simulink model "modelo_geral"  (R2015a)
settings: Solver=ode1  SolverMode=SingleTasking  StartTime=0.0  StopTime=10  FixedStep=0.01  RelTol=1e-3
values from neighbouring files (symbols this model uses):
  K = 54.96    [exp11.m]
  KNL = 59.7881    [exp11.m]
  Kp = 1.604    [exp11.m]
  Kpi = 0.5    [exp11.m]
  Kt = KtL    (= 0.0169213973799)    [exp11.m]
  T = 0.27    [exp11.m]
  U = Kp*pi/2    (= 2.51955730818)    [exp11.m]
undefined symbols (not defined in the file): phi
settings Model: CovExternalEMLEnable=on  Creator=rpm  LastModifiedBy=caiod
settings DataIOCC: LimitDataPoints=off  SignalLoggingSaveFormat=ModelDataLogs  SaveOutput=off  SignalLogging=off  DSMLogging=off  SaveTime=off  TimeSaveName=t
settings OptimizationCC: ExpressionDepthLimit=2147483647  InitFltsAndDblsToZero=on
settings DebuggingCC: UnderspecifiedInitializationDetection=Classic  MergeDetectMultiDrivingBlocksExec=none  FcnCallInpInsideContextMsg=EnableAllAsWarning  StateNameClashWarn=warning
settings GRTTargetCC: CombineOutputUpdateFcns=off  GRTInterface=on

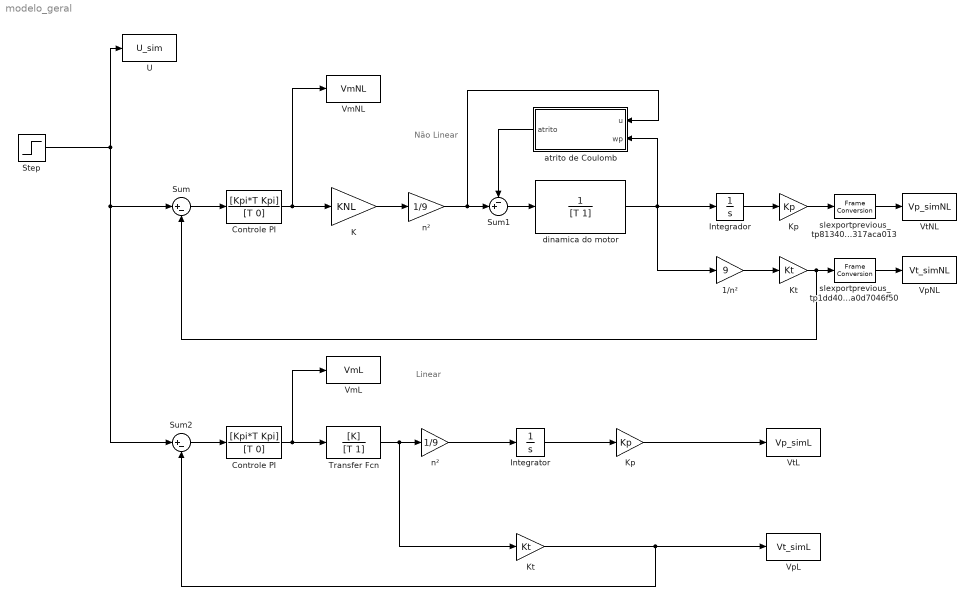
== system modelo_geral ==
  note: Não
      | Linear
  note: Linear
  " VpNL" : ToWorkspace  VariableName=Vt_simNL  SaveFormat=Timeseries  SampleTime=-1
  1/n² : Gain  Gain=9
  Controle PI : TransferFcn  Numerator=[Kpi*T Kpi]  Denominator=[T 0]
  "Controle PI " : TransferFcn  Numerator=[Kpi*T Kpi]  Denominator=[T 0]
  Integrador : Integrator
  Integrator : Integrator
  K : Gain  Gain=KNL
  Kp : Gain  Gain=Kp
  "Kp " : Gain  Gain=Kp
  Kt : Gain  Gain=Kt
  "Kt " : Gain  Gain=Kt
  Step : Step  After=U  SampleTime=0
  Sum : Sum  Inputs=|+-
  Sum1 : Sum  Inputs=-+|
  Sum2 : Sum  Inputs=|+-
  Transfer Fcn : TransferFcn  Numerator=[K]  Denominator=[T 1]
  U : ToWorkspace  VariableName=U_sim  SaveFormat=Timeseries  SampleTime=-1
  "VmL " : ToWorkspace  VariableName=VmL  SaveFormat=Timeseries  SampleTime=-1
  "VmNL " : ToWorkspace  VariableName=VmNL  SaveFormat=Timeseries  SampleTime=-1
  "VpL " : ToWorkspace  VariableName=Vt_simL  SaveFormat=Timeseries  SampleTime=-1
  VtL : ToWorkspace  VariableName=Vp_simL  SaveFormat=Timeseries  SampleTime=-1
  VtNL : ToWorkspace  VariableName=Vp_simNL  SaveFormat=Timeseries  SampleTime=-1
  atrito de Coulomb : Subsystem  mask{phi=phi}
      mask Display: fprintf('phi = %3.1f', phi)
  dinamica do motor : TransferFcn  Denominator=[T 1]
  n² : Gain  Gain=1/9
  "n² " : Gain  Gain=1/9
  slexportprevious_tp1dd40cb0_336a_46da_8b79_bfa0d7046f50 : FrameConversion  OutFrame=Sample-based
  slexportprevious_tp8134031d_9c58_445d_bef1_a0d317aca013 : FrameConversion  OutFrame=Sample-based
  wires:
  dinamica do motor/1 -> 1/n²/1, Integrador/1, atrito de Coulomb/2(wp)
  Integrador/1 -> Kp/1
  K/1 -> n²/1
  n²/1 -> atrito de Coulomb/1(u), Sum1/2
  atrito de Coulomb/1(atrito) -> Sum1/1
  Sum1/1 -> dinamica do motor/1
  1/n²/1 -> Kt/1
  slexportprevious_tp1dd40cb0_336a_46da_8b79_bfa0d7046f50/1 -> " VpNL"/1
  Kp/1 -> slexportprevious_tp8134031d_9c58_445d_bef1_a0d317aca013/1
  slexportprevious_tp8134031d_9c58_445d_bef1_a0d317aca013/1 -> VtNL/1
  Kt/1 -> Sum/2, slexportprevious_tp1dd40cb0_336a_46da_8b79_bfa0d7046f50/1
  Controle PI/1 -> "VmNL "/1, K/1
  Sum/1 -> Controle PI/1
  Sum2/1 -> "Controle PI "/1
  Transfer Fcn/1 -> "Kt "/1, "n² "/1
  "n² "/1 -> Integrator/1
  Integrator/1 -> "Kp "/1
  "Kp "/1 -> VtL/1
  "Kt "/1 -> "VpL "/1, Sum2/2
  Step/1 -> Sum2/1, Sum/1, U/1
  "Controle PI "/1 -> Transfer Fcn/1, "VmL "/1

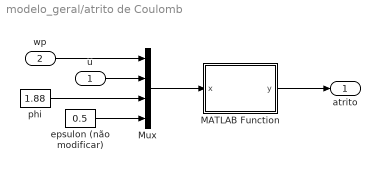
== system modelo_geral/atrito de Coulomb ==
  u : Inport
  wp : Inport  Port=2
  MATLAB Function : MATLAB Function  TreatAsAtomicUnit=on
  Mux : Mux
  epsulon (não modificar) : Constant  Value=0.5
  phi : Constant  Value=1.88
  atrito : Outport
  wires:
  u/1 -> Mux/2
  phi/1 -> Mux/3
  MATLAB Function/1(y) -> atrito/1
  wp/1 -> Mux/1
  epsulon (não modificar)/1 -> Mux/4
  Mux/1 -> MATLAB Function/1(x)

== matlab function modelo_geral/atrito de Coulomb/MATLAB Function ==
  data: x input size=4; y output size=1
function y = nl_coulomb(x)
% Atrito de Coulomb
% Para uso de nl_template.mdl

wp  = x(1); 
u   = x(2); 
phi = x(3); 
epsulon = x(4);

y = 0;

if wp > epsulon
    y = phi;
elseif wp < -epsulon
    y = -phi;
elseif wp >= 0
    y = min(phi,abs(u));
elseif wp < 0
    y = max(-phi,-abs(u));
end
